simulink model "adrc2"  (Simulink 8.9)
settings: Solver=ode45  StartTime=0.0  StopTime=80.0  RelTol=1e-3  EnableMultiTasking=on
settings Model: Creator=admin  LastModifiedBy=admin
settings OptimizationCC: InitFltsAndDblsToZero=on
settings DebuggingCC: SaveWithParameterizedLinksMsg=none  SignalResolutionControl=TryResolveAllWithWarning  SolverPrmCheckMsg=warning  MultiTaskDSMMsg=warning  MultiTaskCondExecSysMsg=none  StateNameClashWarn=none
settings GRTTargetCC: TargetFcnLib=ansi_tfl_tmw.mat  GeneratePreprocessorConditionals=Use local settings

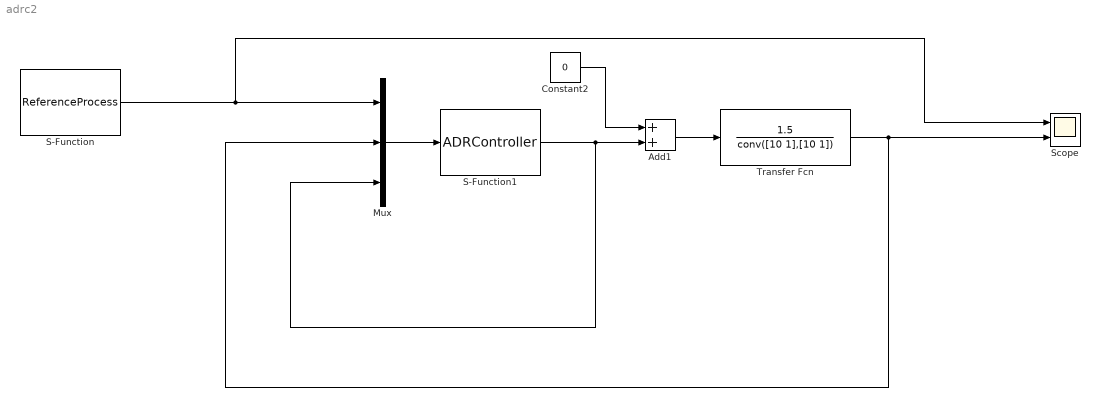
== system adrc2 ==
  Add1 : Sum  SampleTime=0.1
  Constant2 : Constant  Value=0
  Mux : Mux  Inputs=3
  S-Function : S-Function  FunctionName=ReferenceProcess  Parameters=SetPoint, RisingTime,SampleTime  SFunctionDeploymentMode=off  EnableBusSupport=off  mask{SetPoint=1, RisingTime=8, SampleTime=0.1}
  S-Function1 : S-Function  FunctionName=ADRController  Parameters=Beta1,Beta2,Delta1,A1,A2,Delta2,Gamma1,Gamma2,Gamma3,b0,SampleTime  SFunctionDeploymentMode=off  EnableBusSupport=off  mask{Beta1=100, Beta2=80, Delta1=0.2, A1=3/4, A2=3/2, Delta2=0.5, Gamma1=20, Gamma2=20, Gamma3=30, b0=1.5/100, SampleTime=0.1}
      mask prompts: Beta1 "Proportion Coefficient"; Beta2 "Derivation Coefficient"; Delta1 "Linear Region1 of PID"; A1 "Proportion Power"; A2 "Derivation Power"; Delta2 "Linear Region2 of Observer"; Gamma1 "Observer Coefficient1"; Gamma2 "Observer Coefficient2"; Gamma3 "Observer Coefficient3"; b0 "System Gain"; SampleTime "Sample Time"
  Scope : Scope  NumInputPorts=2
  Transfer Fcn : TransferFcn  Numerator=[1.5]  Denominator=conv([10 1],[10 1])
  wires:
  S-Function1/1 -> Mux/3, Add1/2
  Transfer Fcn/1 -> Mux/2, Scope/2
  Mux/1 -> S-Function1/1
  S-Function/1 -> Scope/1, Mux/1
  Constant2/1 -> Add1/1
  Add1/1 -> Transfer Fcn/1
